simulink model "FuncionesDeMembresiaDMA"  (R2024b)
settings: Solver=VariableStepAuto  StartTime=0.0  StopTime=10.0  RelTol=1e-3
settings Model: Creator=david  LastModifiedBy=david

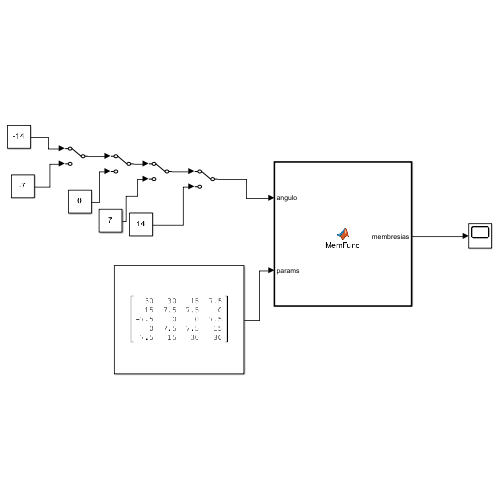
[thumbnail: Simulink's stored preview of the top-level diagram]
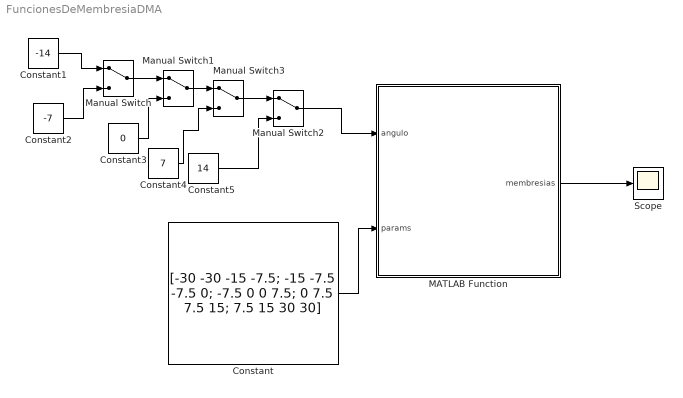
== system FuncionesDeMembresiaDMA ==
  Constant : Constant  Value=[-30 -30 -15 -7.5; -15 -7.5 -7.5 0; -7.5 0 0 7.5; 0 7.5 7.5 15; 7.5 15 30 30]
  Constant1 : Constant  Value=-14
  Constant2 : Constant  Value=-7
  Constant3 : Constant  Value=0
  Constant4 : Constant  Value=7
  Constant5 : Constant  Value=14
  MATLAB Function : MATLAB Function  TreatAsAtomicUnit=on
  Manual Switch{,1..3} (4 alike) : ManualSwitch
  Scope : Scope
  wires:
  Constant/1 -> MATLAB Function/2(params)
  MATLAB Function/1(membresias) -> Scope/1
  Manual Switch/1 -> Manual Switch1/1
  Manual Switch1/1 -> Manual Switch3/1
  Manual Switch3/1 -> Manual Switch2/1
  Manual Switch2/1 -> MATLAB Function/1(angulo)
  Constant5/1 -> Manual Switch2/2
  Constant4/1 -> Manual Switch3/2
  Constant3/1 -> Manual Switch1/2
  Constant2/1 -> Manual Switch/2
  Constant1/1 -> Manual Switch/1

== matlab function FuncionesDeMembresiaDMA/MATLAB Function ==
  data: angulo input; membresias output; params input
function membresias = MemFunc(angulo, params)
% calcular_membresia_flexible: Calcula los valores de membresía para un ángulo
%   dado usando una matriz de parámetros.
%   Input:
%       - angulo: El valor del ángulo (puede ser un escalar o un vector).
%       - params: Una matriz de M x N, donde M es el número de funciones
%                 de membresía y N es el número de parámetros por función.
%                 Formato esperado: [a, b, c, d] para trapezoidal o [a, b, c, c] para triangular.
%   Output:
%       - membresias: Un vector o matriz con los valores de membresía. Cada columna
%                     corresponde a una función de membresía.

% Obtener el número de funciones de membresía de la matriz de parámetros
num_funciones = size(params, 1);

% Inicializar la matriz de resultados. Si angulo es un vector, la matriz de
% resultados tendrá el mismo número de filas que angulo y el número de
% columnas de las funciones.
membresias = zeros(length(angulo), num_funciones);

% Recorrer cada función de membresía definida en la matriz de parámetros
for i = 1:num_funciones
    % Extraer los parámetros de la fila actual
    p = params(i, :);
    
    % Asignar los puntos de control. Si la matriz es 1x3, asumimos que es una triangular.
    if length(p) == 3
        a = p(1);
        b = p(2);
        c = p(3);
        d = p(3); % Para funciones triangulares, c y d son el mismo punto
    elseif length(p) == 4
        a = p(1);
        b = p(2);
        c = p(3);
        d = p(4);
    else
        error('La matriz de parámetros debe tener 3 o 4 columnas.');
    end
    
    % Calcular la membresía para cada ángulo de entrada usando la función 'trapmf'
    % de Fuzzy Logic Toolbox. Esta función puede manejar triángulos y trapezoides.
    % Si no tienes la toolbox, puedes implementar la fórmula manualmente como
    % en la respuesta anterior.
    
    % La siguiente es una implementación manual si no se tiene la toolbox
    mu = zeros(size(angulo));
    
    % Lado izquierdo del trapecio/triángulo
    idx1 = angulo > a & angulo <= b;
    mu(idx1) = (angulo(idx1) - a) / (b - a);
    
    % Parte superior del trapecio (valor 1)
    idx2 = angulo >= b & angulo <= c;
    mu(idx2) = 1;
    
    % Lado derecho del trapecio/triángulo
    idx3 = angulo > c & angulo < d;
    mu(idx3) = (d - angulo(idx3)) / (d - c);
    
    % Asignar el vector de membresía a la columna correspondiente
    membresias(:, i) = mu'; % Transponer si angulo es un vector fila
end

end
